simulink model "sysob_simulink"  (R2019a)
settings: Solver=VariableStepAuto  StartTime=0.0  StopTime=500  MaxStep=.5  RelTol=1e-3
model workspace: external: MAT-File M:\ParaPower\ARL_ParaPower\Validation\MItest.mat (data not in the file)
libraries: simulink x1
settings Model: Creator=michael.c.fish  LastModifiedBy=michael.c.fish
settings DataIOCC: ReturnWorkspaceOutputs=off
settings DebuggingCC: ArithmeticOperatorsInVariantConditions=warning

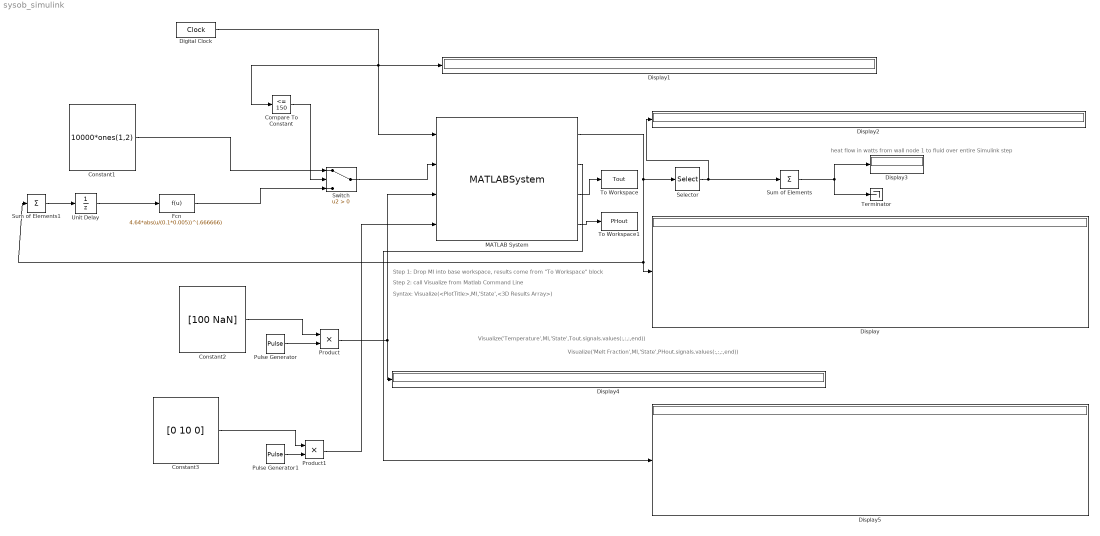
== system sysob_simulink ==
  note: Syntax: Visualize(<PlotTitle>,MI,'State',<3D Results Array>)
  note: Step 2: call Visualize from Matlab Command Line
  note: Step 1: Drop MI into base workspace, results come from "To Workspace" block
  note: Visualize('Temperature',MI,'State',Tout.signals.values(:,:,:,end))
  note: heat flow in watts from wall node 1 to fluid over entire Simulink step
  note: Visualize('Melt Fraction',MI,'State',PHout.signals.values(:,:,:,end))
  Compare To Constant : simulink/Logic and Bit Operations/Compare To Constant  relop=<=  const=150  OutDataTypeStr=boolean
  Constant1 : Constant  Value=10000*ones(1,2)  VectorParams1D=off
  Constant2 : Constant  Value=[100 NaN]  VectorParams1D=off
  Constant3 : Constant  Value=[0 10 0]  VectorParams1D=off
  Digital Clock : DigitalClock  SampleTime=.2
  Display{,1..5} (6 alike) : Display
  Fcn : Fcn  Expr=4.64*abs(u/(0.1*0.005))^(.666666)
  MATLAB System : MATLABSystem  System=hookPPT  MI=MI_CSU  SimulateUsing=Interpreted execution
      mask Type: hookPPT
      mask Display:
      | disp('hookPPT');
      | port_label('input',1,'GlobalTime');
      | port_label('input',2,'htcs');
      | port_label('input',3,'Ta_vec');
      | port_label('input',4,'Q_cmd');
      | port_label('output',1,'bdry_watts');
      | port_label('output',2,'source_temps');
      | port_label('output',3,'Tres');
      | port_label('output',4,'PHres');
  Product : Product
  Product1 : Product
  Pulse Generator : DiscretePulseGenerator  PulseType=Time based  Period=50  PulseWidth=50
  Pulse Generator1 : DiscretePulseGenerator  PulseType=Time based  Period=50  PulseWidth=50
  Selector : Selector  NumberOfDimensions=2  InputPortWidth=3  IndexOptions=Index vector (dialog),Select all  Indices=1,1  OutputSizes=1,1
  Sum of Elements : Sum  Inputs=+
  Sum of Elements1 : Sum  Inputs=+  CollapseMode=Specified dimension
  Switch : Switch  Criteria=u2 > Threshold
  Terminator : Terminator
  To Workspace : ToWorkspace  VariableName=Tout  SaveFormat=Structure With Time  SampleTime=-1
  To Workspace1 : ToWorkspace  VariableName=PHout  SaveFormat=Structure With Time  SampleTime=-1
  Unit Delay : UnitDelay  SampleTime=-1  HasFrameUpgradeWarning=on
  wires:
  MATLAB System/1 -> Sum of Elements1/1, Display/1, Selector/1
  Selector/1 -> Sum of Elements/1, Display2/1
  Pulse Generator/1 -> Product/2
  Constant2/1 -> Product/1
  Product/1 -> MATLAB System/3, Display4/1
  Sum of Elements/1 -> Terminator/1, Display3/1
  Switch/1 -> MATLAB System/2
  Constant1/1 -> Switch/1
  Compare To Constant/1 -> Switch/2
  Unit Delay/1 -> Fcn/1
  Digital Clock/1 -> Compare To Constant/1, MATLAB System/1, Display1/1
  Sum of Elements1/1 -> Unit Delay/1
  Fcn/1 -> Switch/3
  MATLAB System/4 -> To Workspace1/1
  MATLAB System/3 -> To Workspace/1
  MATLAB System/2 -> Display5/1
  Pulse Generator1/1 -> Product1/2
  Constant3/1 -> Product1/1
  Product1/1 -> MATLAB System/4
